simulink model "TPS_FailureDetector"  (R2024b)
settings: Solver=FixedStepDiscrete  StartTime=0.0  StopTime=10.0  FixedStep=1e-1  RelTol=1e-3
settings Model: Creator=MOHAMED  LastModifiedBy=MOHAMED

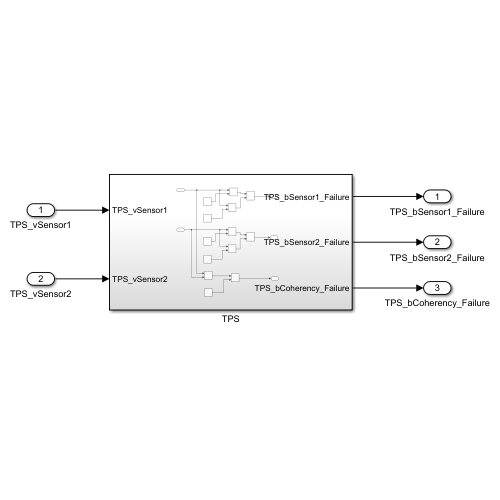
[thumbnail: Simulink's stored preview of the top-level diagram]
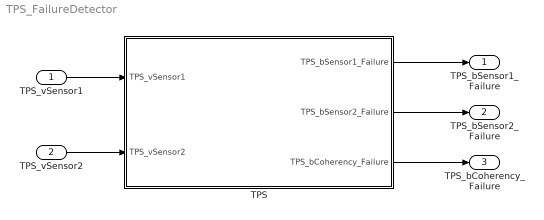
== system TPS_FailureDetector ==
  TPS_vSensor1 : Inport  OutDataTypeStr=single
  TPS_vSensor2 : Inport  Port=2  OutDataTypeStr=single
  TPS : Subsystem
  TPS_bSensor1_Failure : Outport  OutDataTypeStr=boolean
  TPS_bSensor2_Failure : Outport  Port=2  OutDataTypeStr=boolean
  TPS_bCoherency_Failure : Outport  Port=3  OutDataTypeStr=boolean
  wires:
  TPS_vSensor1/1 -> TPS/1(TPS_vSensor1)
  TPS_vSensor2/1 -> TPS/2(TPS_vSensor2)
  TPS/3(TPS_bCoherency_Failure) -> TPS_bCoherency_Failure/1
  TPS/2(TPS_bSensor2_Failure) -> TPS_bSensor2_Failure/1
  TPS/1(TPS_bSensor1_Failure) -> TPS_bSensor1_Failure/1

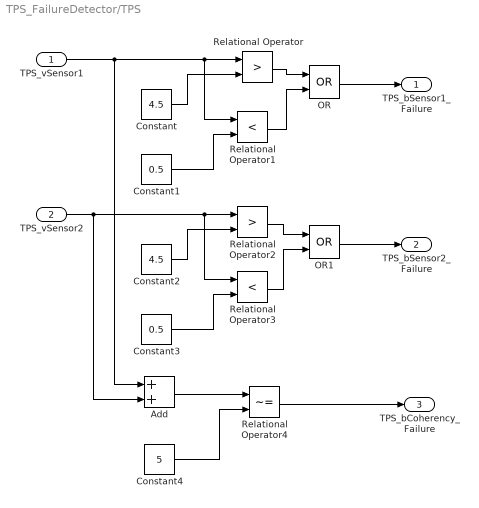
== system TPS_FailureDetector/TPS ==
  TPS_vSensor1 : Inport  OutDataTypeStr=single
  TPS_vSensor2 : Inport  Port=2  OutDataTypeStr=single
  Add : Sum
  Constant : Constant  Value=4.5
  Constant1 : Constant  Value=0.5
  Constant2 : Constant  Value=4.5
  Constant3 : Constant  Value=0.5
  Constant4 : Constant  Value=5
  OR : Logic  Operator=OR  AllPortsSameDT=off  OutDataTypeStr=boolean
  OR1 : Logic  Operator=OR  AllPortsSameDT=off  OutDataTypeStr=boolean
  Relational Operator : RelationalOperator  Operator=>  OutDataTypeStr=boolean  RndMeth=Simplest  InputSameDT=off
  Relational Operator1 : RelationalOperator  Operator=<  OutDataTypeStr=boolean  RndMeth=Simplest  InputSameDT=off
  Relational Operator2 : RelationalOperator  Operator=>  OutDataTypeStr=boolean  RndMeth=Simplest  InputSameDT=off
  Relational Operator3 : RelationalOperator  Operator=<  OutDataTypeStr=boolean  RndMeth=Simplest  InputSameDT=off
  Relational Operator4 : RelationalOperator  Operator=~=  OutDataTypeStr=boolean  RndMeth=Simplest  InputSameDT=off
  TPS_bSensor1_Failure : Outport  OutDataTypeStr=boolean
  TPS_bSensor2_Failure : Outport  Port=2  OutDataTypeStr=boolean
  TPS_bCoherency_Failure : Outport  Port=3  OutDataTypeStr=boolean
  wires:
  Constant/1 -> Relational Operator/2
  Relational Operator1/1 -> OR/2
  Constant2/1 -> Relational Operator2/2
  Constant1/1 -> Relational Operator1/2
  Constant3/1 -> Relational Operator3/2
  TPS_vSensor1/1 -> Add/1, Relational Operator1/1, Relational Operator/1
  TPS_vSensor2/1 -> Relational Operator3/1, Relational Operator2/1, Add/2
  Relational Operator/1 -> OR/1
  OR1/1 -> TPS_bSensor2_Failure/1
  Relational Operator3/1 -> OR1/2
  Relational Operator2/1 -> OR1/1
  OR/1 -> TPS_bSensor1_Failure/1
  Add/1 -> Relational Operator4/1
  Constant4/1 -> Relational Operator4/2
  Relational Operator4/1 -> TPS_bCoherency_Failure/1
